simulink model "q_2dsfl_open_loop"  (R2021a)
settings: Solver=ode1  StartTime=0.0  StopTime=inf  FixedStep=0.002  RelTol=1e-3  EnableMultiTasking=on
values from neighbouring files (symbols this model uses):
  A1 = [0 0 0 0 0 0 628.889014083 -863.33243061 1 0 -62.9562756075 62.9562756075 ... (16 elements, 4x4)]    [lqr_full_10deg.mat]
  A2 = [0 0 0 0 0 0 2271.11688578 -3336.19989408 1 0 -496.762762663 496.762762663 ... (16 elements, 4x4)]    [lqr_full_10deg.mat]
  B1 = [0 0 140.471189949 -140.471189949]    [lqr_full_10deg.mat]
  B2 = [0 0 288.122402345 -288.122402345]    [lqr_full_10deg.mat]
  C1 = [1 0 0 0 0 1 0 0 0 0 1 0 ... (16 elements, 4x4)]    [lqr_full_10deg.mat]
  C2 = [1 0 0 0 0 1 0 0 0 0 1 0 ... (16 elements, 4x4)]    [lqr_full_10deg.mat]
  D1 = [0 0 0 0]    [lqr_full_10deg.mat]
  D2 = [0 0 0 0]    [lqr_full_10deg.mat]
  DTH1_LIM_ENABLE = 1    [lqr_full_10deg.mat]
  DTH2_LIM_ENABLE = 1    [lqr_full_10deg.mat]
  DTH2_MAX = 7.5    [lqr_full_10deg.mat]
  DTH2_MIN = -7.5    [lqr_full_10deg.mat]
  K1_defl_b = 2 / 3 * L1 / T1    [config_2dslf_sensors.m]    (also in lqr_full_10deg.mat = 106.036745407)
  K1_strain_b = 1.286e-4    (= 0.0001286)    [config_2dslf_sensors.m]    (also in lqr_full_10deg.mat)
  K2_defl_b = 2 / 3 * L2 / T2    [config_2dslf_sensors.m]    (also in lqr_full_10deg.mat = 151.368578928)
  K2_strain_b = 1.235e-4    (= 0.0001235)    [config_2dslf_sensors.m]    (also in lqr_full_10deg.mat)
  KE_D1 = K_ENC / Kg1    [config_2dslf_sensors.m]    (also in lqr_full_10deg.mat = 1.53398078789e-05)
  KE_D2 = K_ENC / Kg2    [config_2dslf_sensors.m]    (also in lqr_full_10deg.mat = 3.06796157577e-05)
  LIMIT_SWITCHES_ENABLE = 1    [lqr_full_10deg.mat]
  wcf = 251.327412287    [lqr_full_10deg.mat]
  wcfa = 12.5663706144    [lqr_full_10deg.mat]
  zetaf = 0.9    [lqr_full_10deg.mat]
undefined symbols (not defined in the file or in its folder): HIL, qc_get_step_size
libraries: quarc_library x19, simulink_extras x6
settings Model: SimulationMode=external  ExtModeTrigDuration=60000  Creator=ajavid  LastModifiedBy=hurak
settings SolverCC: AlgebraicLoopSolver=TrustRegion  PositivePriorityOrder=on
settings DataIOCC: LimitDataPoints=on  MaxDataPoints=30000  SaveFormat=Array  SignalLoggingSaveFormat=ModelDataLogs  ReturnWorkspaceOutputs=off
settings OptimizationCC: ExpressionDepthLimit=2147483647  InitFltsAndDblsToZero=on
settings DebuggingCC: SaveWithParameterizedLinksMsg=none  UnderspecifiedInitializationDetection=Classic  MergeDetectMultiDrivingBlocksExec=none  SolverPrmCheckMsg=warning  FcnCallInpInsideContextMsg=warning  StateNameClashWarn=warning  SFUnexpectedBacktrackingDiag=warning  SFNoUnconditionalDefaultTransitionDiag=warning  SFExecutionAtInitializationDiag=none  SFMachineParentedDataDiag=warning  ArithmeticOperatorsInVariantConditions=warning
settings ModelReferenceCC: PropagateSignalLabelsOutOfModel=off
settings RTWCC: Description=QUARC Win64 Target Using Toolchain  SystemTargetFile=quarc_win64.tlc  TemplateMakefile=quarc_default_tmf  Toolchain=QUARC win64 | nmake (64-bit Windows)  BuildConfiguration=Faster Runs
settings CodeAppCC: StateflowObjectComments=on
settings STFCustomTargetCC: ConcurrentExecutionCompliant=on  SystemTargetFile=quarc_win64.tlc
settings GRTTargetCC: TargetLangStandard=C89/C90 (ANSI)  ParMdlRefBuildCompliant=off  CompOptLevelCompliant=off  CombineOutputUpdateFcns=off  MatFileLogging=off  CPPClassGenCompliant=off  GRTInterface=on  ExtMode=on  ExtModeMexFile=quarc_comm
settings ConfigComp: CovMetricSettings=dw  CovSaveCumulativeToWorkspaceVar=on  CovSaveSingleToWorkspaceVar=on

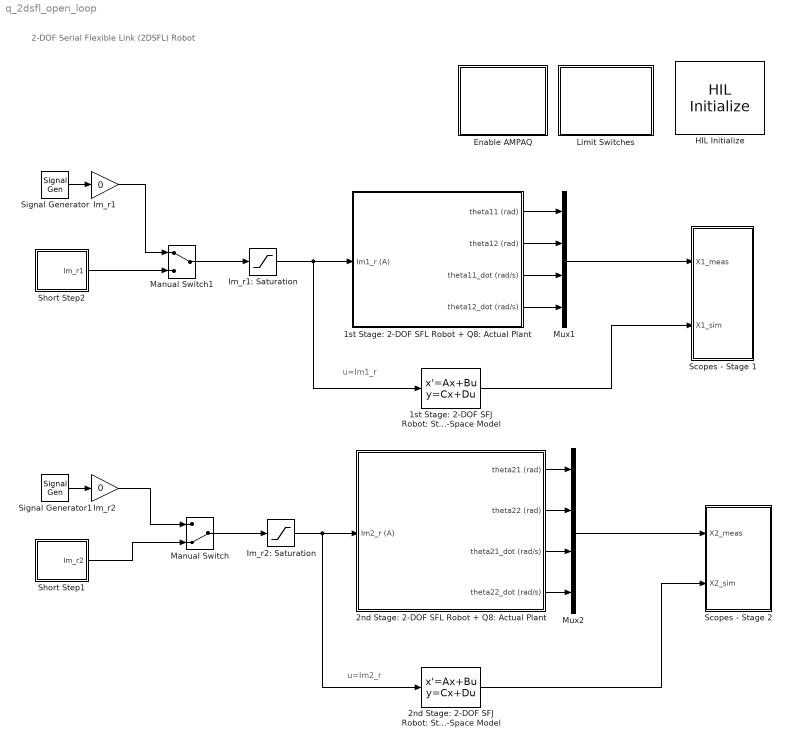
== system q_2dsfl_open_loop ==
  note: 2-DOF Serial Flexible Link (2DSFL) Robot
  note: u=Im1_r
  note: u=Im2_r
  1st Stage: 2-DOF SFJ Robot: State-Space Model : StateSpace  A=A1  B=B1  C=C1  D=D1  InitialCondition=0
  1st Stage: 2-DOF SFL Robot + Q8: Actual Plant : Subsystem
  2nd Stage: 2-DOF SFJ Robot: State-Space Model : StateSpace  A=A2  B=B2  C=C2  D=D2  InitialCondition=0
  2nd Stage: 2-DOF SFL Robot + Q8: Actual Plant : Subsystem
  Enable AMPAQ : Subsystem
  HIL Initialize : quarc_library/Data Acquisition/Generic/Configuration/HIL Initialize  object_name=HIL-1  board_type=q8_usb  board_number=0  board_options=update_rate=normal;decimation=1  exclusive=off  active=on  hardware_clocks=[0:2]  clock_modes=[]  initial_clock_frequencies=[]  set_clock_params_at_start=off  set_clock_params_at_switch_in=off  set_clock_frequencies_at_start=off  set_clock_frequencies_at_switch_in=off  analog_input_channels=[0:7]  analog_input_configurations=[]  analog_input_maximums=10  analog_input_minimums=-10  set_analog_input_params_at_start=on  set_analog_input_params_at_switch_in=off  analog_output_channels=[0:7]  analog_output_maximums=10  analog_output_minimums=-10  initial_analog_outputs=[0]  final_analog_outputs=[0]  watchdog_analog_outputs=0  set_analog_output_params_at_start=on  set_analog_output_params_at_switch_in=off  set_analog_outputs_at_start=on  set_analog_outputs_at_switch_in=off  set_analog_outputs_at_terminate=on  set_analog_outputs_at_switch_out=off  set_analog_outputs_on_watchdog=off  digital_input_channels=[]  digital_output_channels=[]  digital_output_configuration=[]  initial_digital_outputs=[1]  final_digital_outputs=[1]  watchdog_digital_outputs=[1]  set_digital_output_params_at_start=off  set_digital_output_params_at_switch_in=off  set_digital_outputs_at_start=on  set_digital_outputs_at_switch_in=off  set_digital_outputs_at_terminate=on  set_digital_outputs_at_switch_out=off  set_digital_outputs_on_watchdog=off  encoder_channels=[0:7]  quadrature=[4]  encoder_filter_frequency=[]  initial_encoder_counts=[0]  set_encoder_params_at_start=on  set_encoder_params_at_switch_in=off  set_encoder_counts_at_start=on  set_encoder_counts_at_switch_in=off  pwm_channels=[0:7]  pwm_modes=0  pwm_frequency=99.532799999999995e6/4095  pwm_configuration=[0]  pwm_alignment=[0]  pwm_polarity=[1]  pwm_leading_deadband=[0]  pwm_trailing_deadband=[0]  initial_pwm_outputs=[0]  final_pwm_outputs=[0]  watchdog_pwm_outputs=[0]  set_pwm_params_at_start=on  set_pwm_params_at_switch_in=off  set_pwm_outputs_at_start=on  set_pwm_outputs_at_switch_in=off  set_pwm_outputs_at_terminate=on  set_pwm_outputs_at_switch_out=off  set_pwm_outputs_on_watchdog=off  other_output_channels=[]  initial_other_outputs=[]  final_other_outputs=[]  watchdog_other_outputs=[]  set_other_outputs_at_start=off  set_other_outputs_at_switch_in=off  set_other_outputs_at_terminate=off  set_other_outputs_at_switch_out=off  set_other_outputs_on_watchdog=off
  Im_r1 : Gain  Gain=0
  Im_r1: Saturation : Saturate  UpperLimit=0.94  LowerLimit=-0.94
  Im_r2 : Gain  Gain=0
  Im_r2: Saturation : Saturate  UpperLimit=1.2  LowerLimit=-1.2
  Limit Switches : Subsystem
  Manual Switch : ManualSwitch  CurrentSetting=0
  Manual Switch1 : ManualSwitch
  Mux1 : Mux
  Mux2 : Mux
  Scopes - Stage 1 : Subsystem
  Scopes - Stage 2 : Subsystem
  Short Step1 : Subsystem
  Short Step2 : Subsystem
  Signal Generator : SignalGenerator  WaveForm=square
  Signal Generator1 : SignalGenerator  WaveForm=square
  wires:
  1st Stage: 2-DOF SFL Robot + Q8: Actual Plant/3(theta11_dot (rad/s)) -> Mux1/3
  1st Stage: 2-DOF SFJ Robot: State-Space Model/1 -> Scopes - Stage 1/2(X1_sim)
  1st Stage: 2-DOF SFL Robot + Q8: Actual Plant/4(theta12_dot (rad/s)) -> Mux1/4
  1st Stage: 2-DOF SFL Robot + Q8: Actual Plant/2(theta12 (rad)) -> Mux1/2
  1st Stage: 2-DOF SFL Robot + Q8: Actual Plant/1(theta11 (rad)) -> Mux1/1
  Im_r1: Saturation/1 -> 1st Stage: 2-DOF SFL Robot + Q8: Actual Plant/1(Im1_r (A)), 1st Stage: 2-DOF SFJ Robot: State-Space Model/1
  Mux1/1 -> Scopes - Stage 1/1(X1_meas)
  2nd Stage: 2-DOF SFL Robot + Q8: Actual Plant/3(theta21_dot (rad/s)) -> Mux2/3
  2nd Stage: 2-DOF SFJ Robot: State-Space Model/1 -> Scopes - Stage 2/2(X2_sim)
  Mux2/1 -> Scopes - Stage 2/1(X2_meas)
  2nd Stage: 2-DOF SFL Robot + Q8: Actual Plant/4(theta22_dot (rad/s)) -> Mux2/4
  2nd Stage: 2-DOF SFL Robot + Q8: Actual Plant/2(theta22 (rad)) -> Mux2/2
  2nd Stage: 2-DOF SFL Robot + Q8: Actual Plant/1(theta21 (rad)) -> Mux2/1
  Im_r2: Saturation/1 -> 2nd Stage: 2-DOF SFL Robot + Q8: Actual Plant/1(Im2_r (A)), 2nd Stage: 2-DOF SFJ Robot: State-Space Model/1
  Signal Generator/1 -> Im_r1/1
  Signal Generator1/1 -> Im_r2/1
  Manual Switch/1 -> Im_r2: Saturation/1
  Im_r2/1 -> Manual Switch/1
  Im_r1/1 -> Manual Switch1/1
  Manual Switch1/1 -> Im_r1: Saturation/1
  Short Step2/1(Im_r1) -> Manual Switch1/2
  Short Step1/1(Im_r2) -> Manual Switch/2

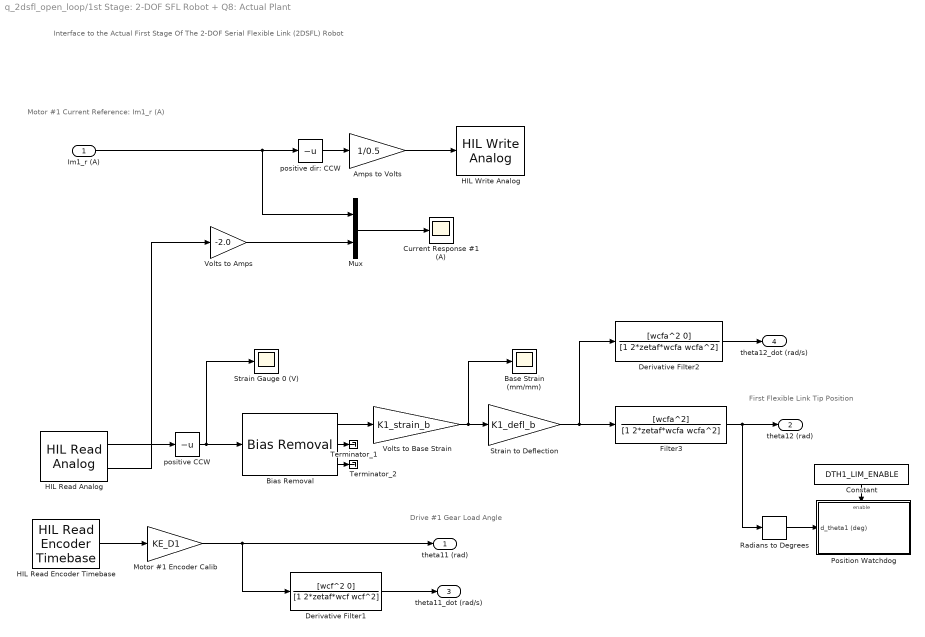
== system q_2dsfl_open_loop/1st Stage: 2-DOF SFL Robot + Q8: Actual Plant ==
  note: Interface to the Actual
      | First Stage Of The 2-DOF Serial Flexible Link (2DSFL) Robot
  note: First Flexible Link
      | Tip Position
  note: Drive #1
      | Gear Load Angle
  note: Motor #1 Current Reference:
      | Im1_r (A)
  Im1_r (A) : Inport
  Amps to Volts : Gain  Gain=1/0.5  SaturateOnIntegerOverflow=on  OutDataTypeStr=Inherit: Same as input  ParamDataTypeStr=Inherit: Same as input
  Base Strain (mm/mm) : Scope
  Bias Removal : quarc_library/Discrete/Bias Removal  start_time=0  end_time=0.2  switch_id=0  sample_time=qc_get_step_size
      settings: SourceProductName=QUARC Targets
  Constant : Constant  Value=DTH1_LIM_ENABLE
  Current Response #1 (A) : Scope
  Derivative Filter1 : TransferFcn  Numerator=[wcf^2 0]  Denominator=[1 2*zetaf*wcf wcf^2]
  Derivative Filter2 : TransferFcn  Numerator=[wcfa^2 0]  Denominator=[1 2*zetaf*wcfa wcfa^2]
  Filter3 : TransferFcn  Numerator=[wcfa^2]  Denominator=[1 2*zetaf*wcfa wcfa^2]
  HIL Read Analog : quarc_library/Data Acquisition/Generic/Immediate I//O/HIL Read Analog  object_name=HIL-1  channels=[0,2]  sample_time=qc_get_step_size  active=on  vector_output=off
  HIL Read Encoder Timebase : quarc_library/Data Acquisition/Generic/Timebases/HIL Read Encoder Timebase  object_name=HIL-1  clock=0  channels=0  active=on  vector_output=off  data_type_mode=Inherit via back propagation  data_type=double  overflow_mode=Error on overflow  samples_in_buffer=max(ceil(1/qc_get_step_size), 1)
  HIL Write Analog : quarc_library/Data Acquisition/Generic/Immediate I//O/HIL Write Analog  object_name=HIL-1  channels=0  sample_time=-1  active=off  vector_input=off
  Motor #1 Encoder Calib : Gain  Gain=KE_D1  SaturateOnIntegerOverflow=on  OutDataTypeStr=Inherit: Same as input  ParamDataTypeStr=Inherit: Same as input
  Mux : Mux  Inputs=2
  Position Watchdog : Subsystem  TreatAsAtomicUnit=on
  Radians to Degrees : simulink_extras/Transformations/Radians to Degrees
  Strain Gauge 0 (V) : Scope
  Strain to Deflection : Gain  Gain=K1_defl_b  SaturateOnIntegerOverflow=on  OutDataTypeStr=Inherit: Same as input  ParamDataTypeStr=Inherit: Same as input
  Terminator_1 : Terminator
  Terminator_2 : Terminator
  Volts to Amps : Gain  Gain=-2.0  OutDataTypeStr=Inherit: Same as input  ParamDataTypeStr=Inherit: Same as input
  Volts to Base Strain : Gain  Gain=K1_strain_b  SaturateOnIntegerOverflow=on  OutDataTypeStr=Inherit: Same as input  ParamDataTypeStr=Inherit: Same as input
  positive CCW : UnaryMinus
  positive dir: CCW : UnaryMinus
  theta11 (rad) : Outport  InitialOutput=0
  theta12 (rad) : Outport  Port=2  InitialOutput=0
  theta11_dot (rad/s) : Outport  Port=3  InitialOutput=0
  theta12_dot (rad/s) : Outport  Port=4  InitialOutput=0
  wires:
  positive CCW/1 -> Bias Removal/1, Strain Gauge 0 (V)/1
  Filter3/1 -> theta12 (rad)/1, Radians to Degrees/1
  Derivative Filter1/1 -> theta11_dot (rad/s)/1
  Derivative Filter2/1 -> theta12_dot (rad/s)/1
  Strain to Deflection/1 -> Filter3/1, Derivative Filter2/1
  Im1_r (A)/1 -> positive dir: CCW/1, Mux/1
  HIL Read Encoder Timebase/1 -> Motor #1 Encoder Calib/1
  Volts to Amps/1 -> Mux/2
  Mux/1 -> Current Response #1 (A)/1
  Motor #1 Encoder Calib/1 -> Derivative Filter1/1, theta11 (rad)/1
  HIL Read Analog/1 -> positive CCW/1
  positive dir: CCW/1 -> Amps to Volts/1
  Volts to Base Strain/1 -> Strain to Deflection/1, Base Strain (mm/mm)/1
  Amps to Volts/1 -> HIL Write Analog/1
  HIL Read Analog/2 -> Volts to Amps/1
  Constant/1 -> Position Watchdog/Enable
  Radians to Degrees/1 -> Position Watchdog/1(d_theta1 (deg))
  Bias Removal/2 -> Terminator_1/1
  Bias Removal/3 -> Terminator_2/1
  Bias Removal/1 -> Volts to Base Strain/1

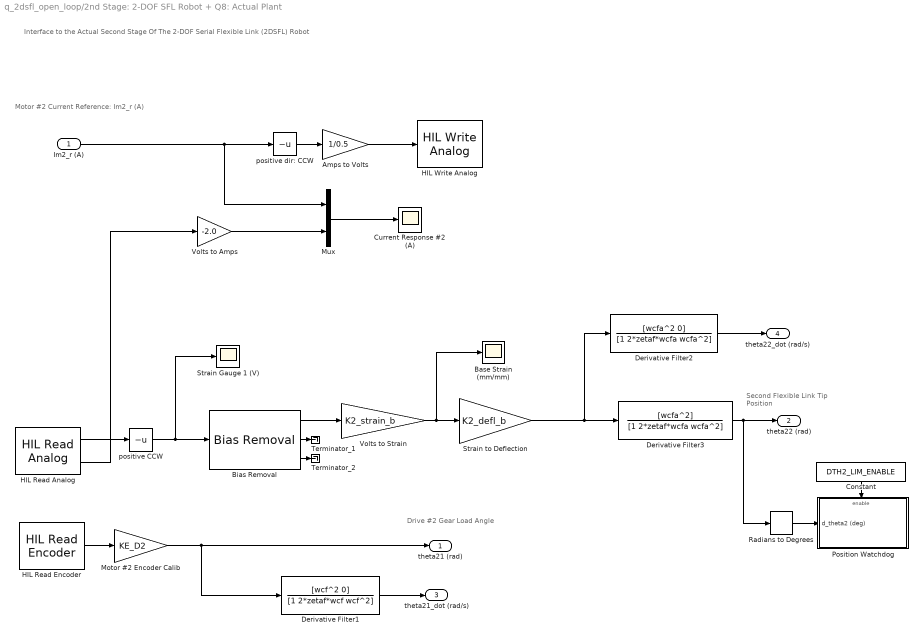
== system q_2dsfl_open_loop/2nd Stage: 2-DOF SFL Robot + Q8: Actual Plant ==
  note: Motor #2 Current Reference:
      | Im2_r (A)
  note: Drive #2
      | Gear Load Angle
  note: Second Flexible Link
      | Tip Position
  note: Interface to the Actual
      | Second Stage Of The 2-DOF Serial Flexible Link (2DSFL) Robot
  Im2_r (A) : Inport
  Amps to Volts : Gain  Gain=1/0.5  SaturateOnIntegerOverflow=on  OutDataTypeStr=Inherit: Same as input  ParamDataTypeStr=Inherit: Same as input
  Base Strain (mm/mm) : Scope
  Bias Removal : quarc_library/Discrete/Bias Removal  start_time=0  end_time=0.2  switch_id=0  sample_time=qc_get_step_size
      settings: SourceProductName=QUARC Targets
  Constant : Constant  Value=DTH2_LIM_ENABLE
  Current Response #2 (A) : Scope
  Derivative Filter1 : TransferFcn  Numerator=[wcf^2 0]  Denominator=[1 2*zetaf*wcf wcf^2]
  Derivative Filter2 : TransferFcn  Numerator=[wcfa^2 0]  Denominator=[1 2*zetaf*wcfa wcfa^2]
  Derivative Filter3 : TransferFcn  Numerator=[wcfa^2]  Denominator=[1 2*zetaf*wcfa wcfa^2]
  HIL Read Analog : quarc_library/Data Acquisition/Generic/Immediate I//O/HIL Read Analog  object_name=HIL-1  channels=[1,3]  sample_time=qc_get_step_size  active=on  vector_output=off
  HIL Read Encoder : quarc_library/Data Acquisition/Generic/Immediate I//O/HIL Read Encoder  object_name=HIL-1  channels=1  sample_time=qc_get_step_size  active=on  vector_output=off  data_type_mode=Inherit via back propagation  data_type=double
  HIL Write Analog : quarc_library/Data Acquisition/Generic/Immediate I//O/HIL Write Analog  object_name=HIL-1  channels=1  sample_time=-1  active=off  vector_input=off
  Motor #2 Encoder Calib : Gain  Gain=KE_D2  SaturateOnIntegerOverflow=on  OutDataTypeStr=Inherit: Same as input  ParamDataTypeStr=Inherit: Same as input
  Mux : Mux  Inputs=2
  Position Watchdog : Subsystem  TreatAsAtomicUnit=on
  Radians to Degrees : simulink_extras/Transformations/Radians to Degrees
  Strain Gauge 1 (V) : Scope
  Strain to Deflection : Gain  Gain=K2_defl_b  SaturateOnIntegerOverflow=on  OutDataTypeStr=Inherit: Same as input  ParamDataTypeStr=Inherit: Same as input
  Terminator_1 : Terminator
  Terminator_2 : Terminator
  Volts to Amps : Gain  Gain=-2.0  OutDataTypeStr=Inherit: Same as input  ParamDataTypeStr=Inherit: Same as input
  Volts to Strain : Gain  Gain=K2_strain_b  SaturateOnIntegerOverflow=on  OutDataTypeStr=Inherit: Same as input  ParamDataTypeStr=Inherit: Same as input
  positive CCW : UnaryMinus
  positive dir: CCW : UnaryMinus
  theta21 (rad) : Outport  InitialOutput=0
  theta22 (rad) : Outport  Port=2  InitialOutput=0
  theta21_dot (rad/s) : Outport  Port=3  InitialOutput=0
  theta22_dot (rad/s) : Outport  Port=4  InitialOutput=0
  wires:
  Derivative Filter3/1 -> theta22 (rad)/1, Radians to Degrees/1
  positive CCW/1 -> Strain Gauge 1 (V)/1, Bias Removal/1
  Derivative Filter2/1 -> theta22_dot (rad/s)/1
  Strain to Deflection/1 -> Derivative Filter3/1, Derivative Filter2/1
  Derivative Filter1/1 -> theta21_dot (rad/s)/1
  Volts to Strain/1 -> Strain to Deflection/1, Base Strain (mm/mm)/1
  HIL Read Analog/1 -> positive CCW/1
  HIL Read Analog/2 -> Volts to Amps/1
  Mux/1 -> Current Response #2 (A)/1
  Volts to Amps/1 -> Mux/2
  HIL Read Encoder/1 -> Motor #2 Encoder Calib/1
  Motor #2 Encoder Calib/1 -> theta21 (rad)/1, Derivative Filter1/1
  Im2_r (A)/1 -> positive dir: CCW/1, Mux/1
  Amps to Volts/1 -> HIL Write Analog/1
  Bias Removal/1 -> Volts to Strain/1
  Constant/1 -> Position Watchdog/Enable
  Radians to Degrees/1 -> Position Watchdog/1(d_theta2 (deg))
  Bias Removal/2 -> Terminator_1/1
  Bias Removal/3 -> Terminator_2/1
  positive dir: CCW/1 -> Amps to Volts/1

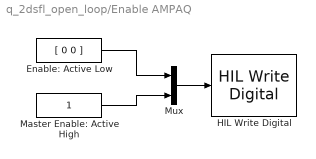
== system q_2dsfl_open_loop/Enable AMPAQ ==
  Enable: Active Low : Constant  Value=[ 0 0 ]
  HIL Write Digital : quarc_library/Data Acquisition/Generic/Immediate I//O/HIL Write Digital  object_name=HIL-1  channels=[0 1 4]  sample_time=-1  active=off  vector_input=on
      settings: SourceProductName=QUARC Targets
  Master Enable: Active High : Constant
  Mux : Mux  Inputs=2
  wires:
  Master Enable: Active High/1 -> Mux/2
  Enable: Active Low/1 -> Mux/1
  Mux/1 -> HIL Write Digital/1

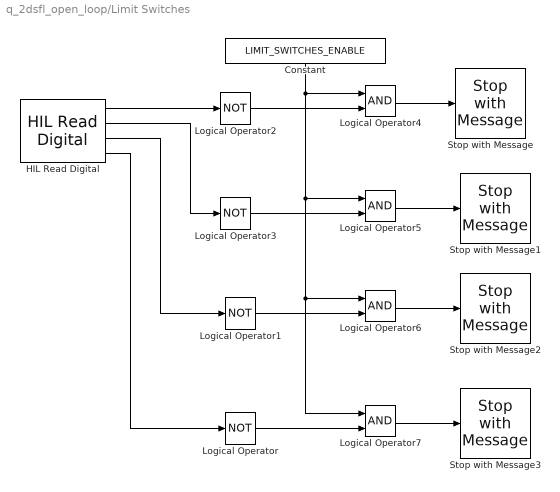
== system q_2dsfl_open_loop/Limit Switches ==
  Constant : Constant  Value=LIMIT_SWITCHES_ENABLE
  HIL Read Digital : quarc_library/Data Acquisition/Generic/Immediate I//O/HIL Read Digital  object_name=HIL-1  channels=[0:3]  sample_time=qc_get_step_size  active=on  vector_output=off  data_type_mode=Inherit via back propagation  data_type=boolean
      settings: AttributesFormatString=(%<object_name>)  SourceProductName=QUARC Targets
  Logical Operator{,1..3} (4 alike) : Logic  Operator=NOT  AllPortsSameDT=off  OutDataTypeStr=boolean
  Logical Operator{4..7} (4 alike) : Logic  AllPortsSameDT=off  OutDataTypeStr=boolean
  Stop with Message : quarc_library/Sinks/Error Handling/Stop with Message  message_type=Fixed error message  message_icon=Error  message=STAGE 1: MAX limit switch hit.
  Stop with Message1 : quarc_library/Sinks/Error Handling/Stop with Message  message_type=Fixed error message  message_icon=Error  message=STAGE 1: MIN limit switch hit.
  Stop with Message2 : quarc_library/Sinks/Error Handling/Stop with Message  message_type=Fixed error message  message_icon=Error  message=STAGE 2: MAX limit switch hit.
  Stop with Message3 : quarc_library/Sinks/Error Handling/Stop with Message  message_type=Fixed error message  message_icon=Error  message=STAGE 2: MIN limit switch hit.
  wires:
  Logical Operator7/1 -> Stop with Message3/1
  Logical Operator6/1 -> Stop with Message2/1
  Logical Operator5/1 -> Stop with Message1/1
  Logical Operator4/1 -> Stop with Message/1
  HIL Read Digital/4 -> Logical Operator/1
  HIL Read Digital/3 -> Logical Operator1/1
  HIL Read Digital/2 -> Logical Operator3/1
  HIL Read Digital/1 -> Logical Operator2/1
  Logical Operator2/1 -> Logical Operator4/2
  Constant/1 -> Logical Operator4/1, Logical Operator5/1, Logical Operator6/1, Logical Operator7/1
  Logical Operator3/1 -> Logical Operator5/2
  Logical Operator1/1 -> Logical Operator6/2
  Logical Operator/1 -> Logical Operator7/2

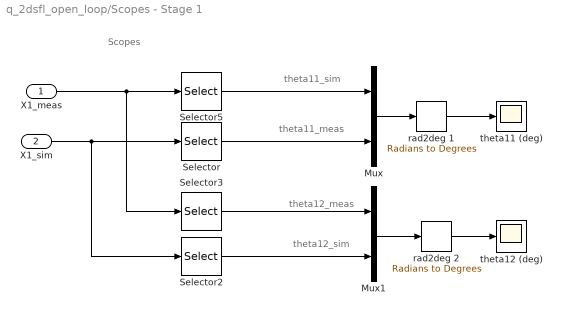
== system q_2dsfl_open_loop/Scopes - Stage 1 ==
  note: Scopes
  note: theta12_sim
  note: theta11_sim
  note: theta11_meas
  note: theta12_meas
  X1_meas : Inport
  X1_sim : Inport  Port=2
  Mux : Mux  Inputs=2
  Mux1 : Mux  Inputs=2
  Selector : Selector  InputPortWidth=4  IndexOptions=Index vector (dialog)  Indices=[1]  OutputSizes=1
  Selector2 : Selector  InputPortWidth=4  IndexOptions=Index vector (dialog)  Indices=[2]  OutputSizes=1
  Selector3 : Selector  InputPortWidth=4  IndexOptions=Index vector (dialog)  Indices=[2]  OutputSizes=1
  Selector5 : Selector  InputPortWidth=4  IndexOptions=Index vector (dialog)  Indices=[1]  OutputSizes=1
  rad2deg 1 : simulink_extras/Transformations/Radians to Degrees
  rad2deg 2 : simulink_extras/Transformations/Radians to Degrees
  theta11 (deg) : Scope
  theta12 (deg) : Scope
  wires:
  X1_meas/1 -> Selector3/1, Selector5/1
  Mux/1 -> rad2deg 1/1
  Mux1/1 -> rad2deg 2/1
  X1_sim/1 -> Selector/1, Selector2/1
  rad2deg 1/1 -> theta11 (deg)/1
  rad2deg 2/1 -> theta12 (deg)/1
  Selector5/1 -> Mux/1
  Selector/1 -> Mux/2
  Selector2/1 -> Mux1/2
  Selector3/1 -> Mux1/1

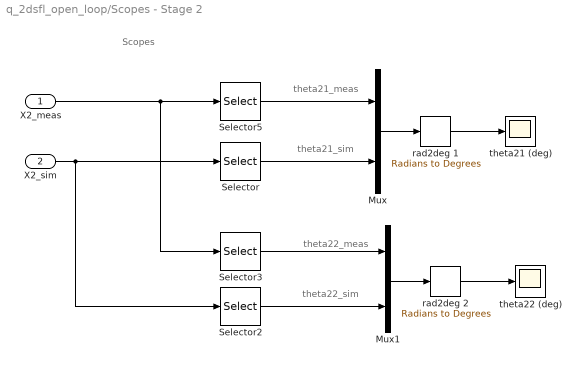
== system q_2dsfl_open_loop/Scopes - Stage 2 ==
  note: Scopes
  note: theta22_sim
  note: theta21_sim
  note: theta21_meas
  note: theta22_meas
  X2_meas : Inport
  X2_sim : Inport  Port=2
  Mux : Mux  Inputs=2
  Mux1 : Mux  Inputs=2
  Selector : Selector  InputPortWidth=4  IndexOptions=Index vector (dialog)  Indices=[1]  OutputSizes=1
  Selector2 : Selector  InputPortWidth=4  IndexOptions=Index vector (dialog)  Indices=[2]  OutputSizes=1
  Selector3 : Selector  InputPortWidth=4  IndexOptions=Index vector (dialog)  Indices=[2]  OutputSizes=1
  Selector5 : Selector  InputPortWidth=4  IndexOptions=Index vector (dialog)  Indices=[1]  OutputSizes=1
  rad2deg 1 : simulink_extras/Transformations/Radians to Degrees
  rad2deg 2 : simulink_extras/Transformations/Radians to Degrees
  theta21 (deg) : Scope
  theta22 (deg) : Scope
  wires:
  Mux/1 -> rad2deg 1/1
  Mux1/1 -> rad2deg 2/1
  X2_meas/1 -> Selector3/1, Selector5/1
  X2_sim/1 -> Selector2/1, Selector/1
  rad2deg 1/1 -> theta21 (deg)/1
  rad2deg 2/1 -> theta22 (deg)/1
  Selector3/1 -> Mux1/1
  Selector2/1 -> Mux1/2
  Selector5/1 -> Mux/1
  Selector/1 -> Mux/2

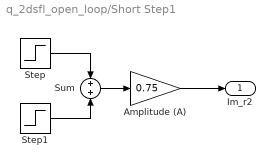
== system q_2dsfl_open_loop/Short Step1 ==
  Amplitude (A) : Gain  Gain=0.75
  Step : Step  SampleTime=0
  Step1 : Step  Time=1.2  After=-1  SampleTime=0
  Sum : Sum
  Im_r2 : Outport
  wires:
  Sum/1 -> Amplitude (A)/1
  Step1/1 -> Sum/2
  Step/1 -> Sum/1
  Amplitude (A)/1 -> Im_r2/1

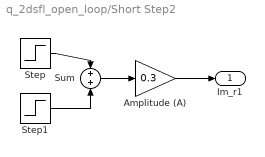
== system q_2dsfl_open_loop/Short Step2 ==
  Amplitude (A) : Gain  Gain=0.3
  Step : Step  SampleTime=0
  Step1 : Step  Time=1.2  After=-1  SampleTime=0
  Sum : Sum
  Im_r1 : Outport
  wires:
  Amplitude (A)/1 -> Im_r1/1
  Step/1 -> Sum/1
  Step1/1 -> Sum/2
  Sum/1 -> Amplitude (A)/1

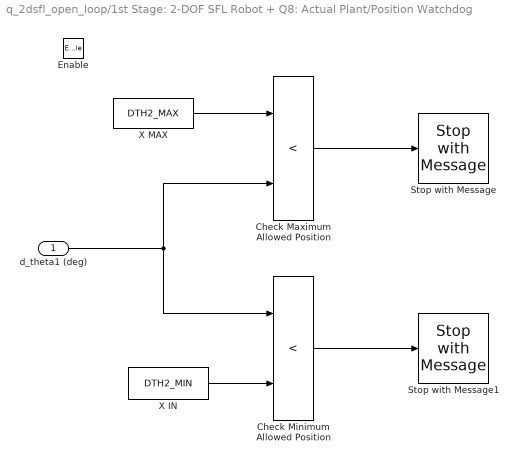
== system q_2dsfl_open_loop/1st Stage: 2-DOF SFL Robot + Q8: Actual Plant/Position Watchdog ==
  d_theta1 (deg) : Inport
  Enable : EnablePort
  Check Maximum Allowed Position : RelationalOperator  Operator=<  RndMeth=Nearest  InputSameDT=on
  Check Minimum Allowed Position : RelationalOperator  Operator=<  RndMeth=Nearest  InputSameDT=on
  Stop with Message : quarc_library/Sinks/Error Handling/Stop with Message  message_type=Fixed error message  message_icon=Error  message=Stage 1 link went above DTH1_MAX variable.
  Stop with Message1 : quarc_library/Sinks/Error Handling/Stop with Message  message_type=Fixed error message  message_icon=Error  message=Stage 1 link went below DTH1_MIN variable.
  X IN : Constant  Value=DTH2_MIN
  X MAX : Constant  Value=DTH2_MAX
  wires:
  d_theta1 (deg)/1 -> Check Minimum Allowed Position/1, Check Maximum Allowed Position/2
  X IN/1 -> Check Minimum Allowed Position/2
  X MAX/1 -> Check Maximum Allowed Position/1
  Check Maximum Allowed Position/1 -> Stop with Message/1
  Check Minimum Allowed Position/1 -> Stop with Message1/1

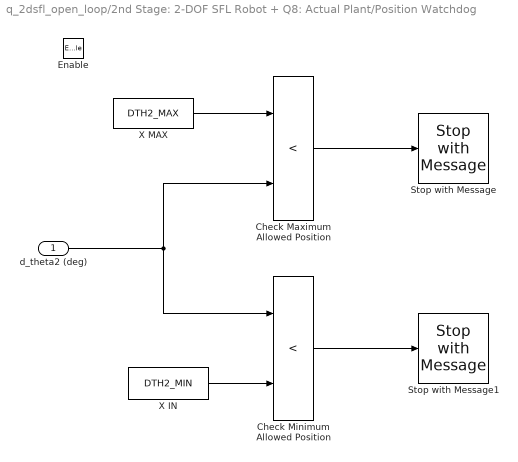
== system q_2dsfl_open_loop/2nd Stage: 2-DOF SFL Robot + Q8: Actual Plant/Position Watchdog ==
  d_theta2 (deg) : Inport
  Enable : EnablePort
  Check Maximum Allowed Position : RelationalOperator  Operator=<  RndMeth=Nearest  InputSameDT=on
  Check Minimum Allowed Position : RelationalOperator  Operator=<  RndMeth=Nearest  InputSameDT=on
  Stop with Message : quarc_library/Sinks/Error Handling/Stop with Message  message_type=Fixed error message  message_icon=Error  message=Stage 2 link went above DTH2_MAX variable.
  Stop with Message1 : quarc_library/Sinks/Error Handling/Stop with Message  message_type=Fixed error message  message_icon=Error  message=Stage 2 link went below DTH2_MIN variable.
  X IN : Constant  Value=DTH2_MIN
  X MAX : Constant  Value=DTH2_MAX
  wires:
  d_theta2 (deg)/1 -> Check Minimum Allowed Position/1, Check Maximum Allowed Position/2
  X IN/1 -> Check Minimum Allowed Position/2
  X MAX/1 -> Check Maximum Allowed Position/1
  Check Maximum Allowed Position/1 -> Stop with Message/1
  Check Minimum Allowed Position/1 -> Stop with Message1/1
